simulink model "DP_GAp"  (R2023b)
settings: Solver=ode45  StartTime=0.0  StopTime=1500  RelTol=1e-3  EnableMultiTasking=on
undefined symbols (not defined in the file or in its folder): Als, Ats, Loa, pa, Ta_p
libraries: simulink x7, simulink_extras x4, marine_gnc x4, slpidlib x2
settings Model: Creator=Lenovo  LastModifiedBy=Ly Soi
settings SolverCC: AlgebraicLoopSolver=TrustRegion
settings DataIOCC: LimitDataPoints=on  SaveFormat=Array  SignalLoggingSaveFormat=ModelDataLogs  ReturnWorkspaceOutputs=off  SignalLoggingName=sigsOut
settings OptimizationCC: InitFltsAndDblsToZero=on  LifeSpan=inf
settings DebuggingCC: SaveWithParameterizedLinksMsg=none  UnderspecifiedInitializationDetection=Classic  MergeDetectMultiDrivingBlocksExec=none  SignalResolutionControl=TryResolveAllWithWarning  MultiTaskDSMMsg=warning  MultiTaskCondExecSysMsg=none  FcnCallInpInsideContextMsg=warning  UnconnectedInputMsg=warning  UnconnectedOutputMsg=warning  UnconnectedLineMsg=warning  SFUnexpectedBacktrackingDiag=warning  SFNoUnconditionalDefaultTransitionDiag=warning  ArithmeticOperatorsInVariantConditions=warning
settings HardwareCC: ProdBitPerPointer=32  ProdBitPerSizeT=32  ProdBitPerPtrDiffT=32  ProdLargestAtomicFloat=None  ProdIntDivRoundTo=Undefined  ProdEndianess=Unspecified  ProdWordSize=32  ProdHWDeviceType=32-bit Generic  TargetUnknown=on
settings ModelReferenceCC: EnableRefExpFcnMdlSchedulingChecks=on  PropagateSignalLabelsOutOfModel=off
settings SFSimCC: SimUseLocalCustomCode=off  CustomCodeUndefinedFunction=UseInterfaceOnly
settings RTWCC: RTWUseLocalCustomCode=off
settings CodeAppCC: StateflowObjectComments=on
settings GRTTargetCC: TargetFcnLib=ansi_tfl_tmw.mat  TargetLangStandard=C89/C90 (ANSI)  ModelReferenceCompliant=off  CombineOutputUpdateFcns=off  MatFileLogging=off  GRTInterface=on
settings ConfigComp: CovMetricSettings=dw  CovSaveCumulativeToWorkspaceVar=on  CovSaveSingleToWorkspaceVar=on  CovExternalEMLEnable=off  CovSFcnEnable=off

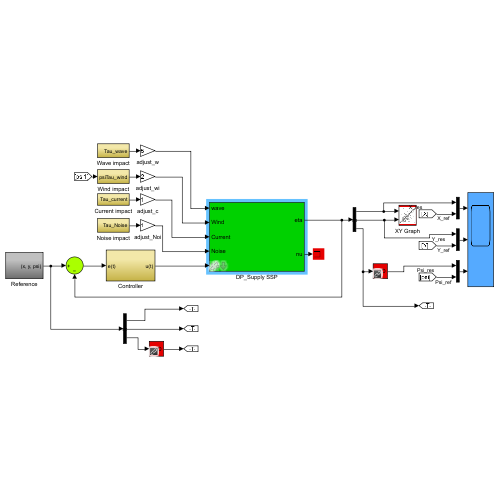
[thumbnail: Simulink's stored preview of the top-level diagram]
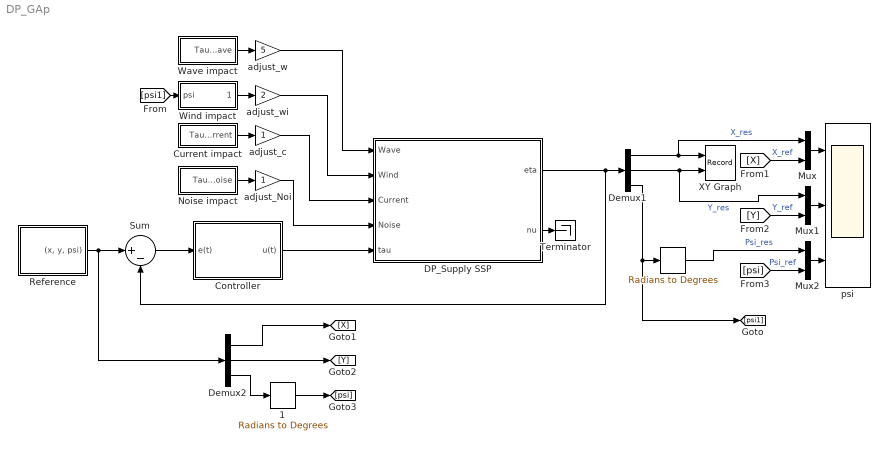
== system DP_GAp ==
  "    " : simulink_extras/Transformations/Radians to Degrees
  "    1" : simulink_extras/Transformations/Radians to Degrees
  Controller : Subsystem
  Current impact : Subsystem
  DP_Supply SSP : Subsystem  AncestorBlock=marine_gnc/Examples/Vessels/Supply vessel  mask(Supply Vessel (surge, sway and yaw)){D=[5.0242e4 0 0; 0 2.7229e5 -4.3933e6; 0 -4.3933e6 4.1894e8], Minv=inv( [5.3122e6 0 0; 0 8.2831e6 0; 0 0 3.7454e9] )}
      mask prompts: D "Linear damping matrix: D"; Minv "Inverse inertia matrix: Minv"
      mask help:
      | DP model
      |
      | Inputs:
      |
      |    tau = 3 DOF control input vector (generalized force)
      |
      | Outputs:
      |
      |    eta = [x, y, psi]'
      |    nu  = [u, v, r]'
      mask Display:
      | color('black'); port_label('output', 1, 'eta')
      | color('black'); port_label('output', 2, 'nu')
      | color('black'); port_label('input', 1, 'wave')
      | color('black'); port_label('input', 2, 'Wind')
      | color('black'); port_label('input', 3, 'Current')
      | color('black'); port_label('input', 4, 'Noise')
      | color('black'); port_label('input', 5, 'tau')
  Demux1 : Demux  Outputs=3
      settings: DisplayOption=none
  Demux2 : Demux  Outputs=3
      settings: DisplayOption=none
  Mux : Mux  Inputs=2
  Mux1 : Mux  Inputs=2
  Mux2 : Mux  Inputs=2
  Noise impact : Subsystem
  Reference : Subsystem
  Sum : Sum  Inputs=|+-
  Terminator : Terminator
  Wave impact : Subsystem
  Wind impact : Subsystem
  XY Graph : Record  FileSettingsInternal="{\"entries\":[{\"content\":{\"excelSettings\":{\"content\":{},\"type\":\"Streamout.ExcelSettings\"}},\"type\":\"Streamout.FileSettingStorage\",\"uuid\":\"\"}],\"packageUris\":[\"http:\\/\\/schema.mathworks.com\\/mf0\\/streamout_blocks\\/R2020a\"],\"version\":\"1.0\"}"  Layout=[1 1]  SignalsInternal="{\"entries\":[{\"content\":{\"signals\":[{\"content\":{\"blockPath\":[],\"dimensions\":[1],\"domain\":\"\",\"lineColor\":\"#a2142f\",\"plots\":[1],\"port\":1,\"signalID\":8,\"signalName\":\"XY Graph:1\"},\"type\":\"RecordBlkView.Signal\",\"uuid\":\"\"},{\"content\":{\"blockPath\":[],\"dimensions\":[1],\"domain\":\"\",\"lineColor\":\"#139fff\",\"plots\":[1],\"port\":2,\"signalID\":11,\"signalName\":\"XY Graph:2\"},\"type\":\"RecordBlkView.Signal\",\"uuid\":\"\"}]},\"type\":\"RecordBlkView.InputSignals\",\"uuid\":\"\"}],\"packageUris\":[\"http:\\/\\/schema.mathworks.com\\/mf0\\/streamout_blocks\\/R2020a\"],\"version\":\"1.0\"}"  VisualizationBindings="{\"xyplotplugin\":{\"info\":[{\"series\":[{\"bindingParametersList\":[{\"parameter\":\"X-Axis\",\"signalID\":8,\"signalName\":\"XY Graph:1\"},{\"parameter\":\"Y-Axis\",\"signalID\":11,\"signalName\":\"XY Graph:2\"}],\"seriesID\":17688}],\"subplotID\":1}]}}"  CompatibilityTag=XY  st=0.1
  adjust_Noi : Gain
  adjust_c : Gain
  adjust_w : Gain  Gain=5
  adjust_wi : Gain  Gain=2
  psi : Scope  NumInputPorts=3
  wires:
  Reference/1("(x, y, psi)") -> Demux2/1, Sum/1
  Sum/1 -> Controller/1(e(t))
  DP_Supply SSP/2(nu) -> Terminator/1
  Demux1/1 -> Mux/1, XY Graph/1  "X_res"
  Demux1/2 -> Mux1/1, XY Graph/2  "Y_res"
  DP_Supply SSP/1(eta) -> Sum/2, Demux1/1
  Demux1/3 -> "    "/1, [psi1]
  Controller/1(u(t)) -> DP_Supply SSP/5(tau)
  Mux/1 -> psi/1
  [X] -> Mux/2  "X_ref"
  Demux2/1 -> [X]
  Mux1/1 -> psi/2
  [Y] -> Mux1/2  "Y_ref"
  Demux2/2 -> [Y]
  Mux2/1 -> psi/3
  [psi] -> Mux2/2  "Psi_ref"
  "    "/1 -> Mux2/1  "Psi_res"
  Demux2/3 -> "    1"/1
  "    1"/1 -> [psi]
  Current impact/1(Tau_current) -> adjust_c/1
  Wave impact/1(Tau_wave) -> adjust_w/1
  Noise impact/1(Tau_Noise) -> adjust_Noi/1
  Wind impact/1(Tau_wind) -> adjust_wi/1
  [psi1] -> Wind impact/1(psi)
  adjust_Noi/1 -> DP_Supply SSP/4(Noise)
  adjust_c/1 -> DP_Supply SSP/3(Current)
  adjust_wi/1 -> DP_Supply SSP/2(Wind)
  adjust_w/1 -> DP_Supply SSP/1(Wave)

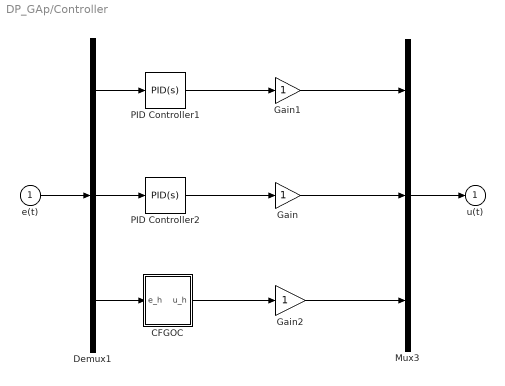
== system DP_GAp/Controller ==
  e(t) : Inport
  CFGOC : Subsystem
  Demux1 : Demux  Outputs=3
  Gain : Gain
  Gain1 : Gain
  Gain2 : Gain
  Mux3 : Mux  Inputs=3
  PID Controller1 : slpidlib/PID Controller  Controller=PID  Form=Parallel  TimeDomain=Continuous-time  UseExternalTs=off  SampleTime=-1  IntegratorMethod=Forward Euler  FilterMethod=Forward Euler  ControllerParametersSource=internal  P=13982.7626612688  I=79.4713079858411  UseKiTs=off  D=614214.172913347  N=13.3180631687176  UseFilter=on  TunerSelectOption=Transfer Function Based (PID Tuner App)  InitialConditionSource=internal  InitialConditionForIntegrator=0  InitialConditionForFilter=0  DifferentiatorICPrevScaledInput=0  ExternalReset=none  TrackingMode=off  Kt=1  LimitOutput=off  SatLimitsSource=internal  UpperSaturationLimit=inf  LowerSaturationLimit=-inf  LinearizeAsGain=on  AntiWindupMode=none  Kb=1  LimitIntegrator=off  UpperIntegratorSaturationLimit=inf  LowerIntegratorSaturationLimit=-inf  POutMin=[]  POutMax=[]  IOutMin=[]  IOutMax=[]  DOutMin=[]  DOutMax=[]  NOutMin=[]  NOutMax=[]  SumOutMin=[]  SumOutMax=[]  SaturationOutMin=[]  SaturationOutMax=[]  PParamMin=[]  PParamMax=[]  IParamMin=[]  IParamMax=[]  DParamMin=[]  DParamMax=[]  NParamMin=[]  NParamMax=[]  KbParamMin=[]  KbParamMax=[]  KtParamMin=[]  KtParamMax=[]  KbOutMin=[]  KbOutMax=[]  KtOutMin=[]  KtOutMax=[]  IntegratorOutMin=[]  IntegratorOutMax=[]  FilterOutMin=[]  FilterOutMax=[]  SumI1OutMin=[]  SumI1OutMax=[]  SumI2OutMin=[]  SumI2OutMax=[]  SumI3OutMin=[]  SumI3OutMax=[]  SumI4OutMin=[]  SumI4OutMax=[]  SumDOutMin=[]  SumDOutMax=[]  DifferentiatorOutMin=[]  DifferentiatorOutMax=[]  FilterDiffOutCoefMin=[]  FilterDiffOutCoefMax=[]  ReciprocalOutMin=[]  ReciprocalOutMax=[]  SumDenOutMin=[]  SumDenOutMax=[]  SumNumOutMin=[]  SumNumOutMax=[]  DivideOutMin=[]  DivideOutMax=[]  UdiffTsProdOutMin=[]  UdiffTsProdOutMax=[]  NTsProdOutMin=[]  NTsProdOutMax=[]  UintegralTsProdOutMin=[]  UintegralTsProdOutMax=[]  UngainTsProdOutMin=[]  UngainTsProdOutMax=[]  ClampingZeroOutDataTypeStr=Inherit: Inherit via back propagation  ClampingZeroOutMin=[]  ClampingZeroOutMax=[]  FilterDenConstantOutDataTypeStr=Inherit: Inherit via back propagation  FilterDenConstantOutMin=[]  FilterDenConstantOutMax=[]  PCopyOutDataTypeStr=Inherit: Inherit via back propagation  PCopyOutMin=[]  PCopyOutMax=[]  NCopyOutDataTypeStr=Inherit: Inherit via back propagation  NCopyOutMin=[]  NCopyOutMax=[]  IntegratorContinuousStateAttributes=''  IntegratorStateMustResolveToSignalObject=off  IntegratorRTWStateStorageClass=Auto  FilterContinuousStateAttributes=''  FilterStateMustResolveToSignalObject=off  FilterRTWStateStorageClass=Auto  ParallelPVariant=InternalParameters  IdealPVariant=Disabled  IVariant=InternalParameters  DVariant=InternalParameters  IntegratorVariant=Continuous  SatVariant=Disabled  AWVariant=Passthrough  PCopyVariant=Disabled  TRVariant=Disabled  FdbkBlocksVariant=Forward  IdealPFdbkVariant=Disabled  SatFdbkVariant=Disabled  DerivativeFilterVariant=ContFilter  NVariant=InternalParameters  NCopyVariant=Disabled  FilterICVariant=InternalICsFilter  IntegratorICVariant=InternalICs  ExternalResetVariant=Disabled  TRSumVariant=Passthrough  SumFdbkVariant=Disabled  SumVariant=Sum_PID  TsampFilterVariant=InternalTs  TsampNgainVariant=Passthrough  TsampIntegralVariant=Disabled_SignalSpec  ExternalSaturationOutDataTypeStr=Inherit: Same as second input
  PID Controller2 : slpidlib/PID Controller  Controller=PID  Form=Parallel  TimeDomain=Continuous-time  UseExternalTs=off  SampleTime=-1  IntegratorMethod=Forward Euler  FilterMethod=Forward Euler  ControllerParametersSource=internal  P=330751.15042107  I=6499.51593881031  UseKiTs=off  D=3225830.41285156  N=4.23253792984163  UseFilter=on  TunerSelectOption=Transfer Function Based (PID Tuner App)  InitialConditionSource=internal  InitialConditionForIntegrator=0  InitialConditionForFilter=0  DifferentiatorICPrevScaledInput=0  ExternalReset=none  TrackingMode=off  Kt=1  LimitOutput=off  SatLimitsSource=internal  UpperSaturationLimit=inf  LowerSaturationLimit=-inf  LinearizeAsGain=on  AntiWindupMode=none  Kb=1  LimitIntegrator=off  UpperIntegratorSaturationLimit=inf  LowerIntegratorSaturationLimit=-inf  POutMin=[]  POutMax=[]  IOutMin=[]  IOutMax=[]  DOutMin=[]  DOutMax=[]  NOutMin=[]  NOutMax=[]  SumOutMin=[]  SumOutMax=[]  SaturationOutMin=[]  SaturationOutMax=[]  PParamMin=[]  PParamMax=[]  IParamMin=[]  IParamMax=[]  DParamMin=[]  DParamMax=[]  NParamMin=[]  NParamMax=[]  KbParamMin=[]  KbParamMax=[]  KtParamMin=[]  KtParamMax=[]  KbOutMin=[]  KbOutMax=[]  KtOutMin=[]  KtOutMax=[]  IntegratorOutMin=[]  IntegratorOutMax=[]  FilterOutMin=[]  FilterOutMax=[]  SumI1OutMin=[]  SumI1OutMax=[]  SumI2OutMin=[]  SumI2OutMax=[]  SumI3OutMin=[]  SumI3OutMax=[]  SumI4OutMin=[]  SumI4OutMax=[]  SumDOutMin=[]  SumDOutMax=[]  DifferentiatorOutMin=[]  DifferentiatorOutMax=[]  FilterDiffOutCoefMin=[]  FilterDiffOutCoefMax=[]  ReciprocalOutMin=[]  ReciprocalOutMax=[]  SumDenOutMin=[]  SumDenOutMax=[]  SumNumOutMin=[]  SumNumOutMax=[]  DivideOutMin=[]  DivideOutMax=[]  UdiffTsProdOutMin=[]  UdiffTsProdOutMax=[]  NTsProdOutMin=[]  NTsProdOutMax=[]  UintegralTsProdOutMin=[]  UintegralTsProdOutMax=[]  UngainTsProdOutMin=[]  UngainTsProdOutMax=[]  ClampingZeroOutDataTypeStr=Inherit: Inherit via back propagation  ClampingZeroOutMin=[]  ClampingZeroOutMax=[]  FilterDenConstantOutDataTypeStr=Inherit: Inherit via back propagation  FilterDenConstantOutMin=[]  FilterDenConstantOutMax=[]  PCopyOutDataTypeStr=Inherit: Inherit via back propagation  PCopyOutMin=[]  PCopyOutMax=[]  NCopyOutDataTypeStr=Inherit: Inherit via back propagation  NCopyOutMin=[]  NCopyOutMax=[]  IntegratorContinuousStateAttributes=''  IntegratorStateMustResolveToSignalObject=off  IntegratorRTWStateStorageClass=Auto  FilterContinuousStateAttributes=''  FilterStateMustResolveToSignalObject=off  FilterRTWStateStorageClass=Auto  ParallelPVariant=InternalParameters  IdealPVariant=Disabled  IVariant=InternalParameters  DVariant=InternalParameters  IntegratorVariant=Continuous  SatVariant=Disabled  AWVariant=Passthrough  PCopyVariant=Disabled  TRVariant=Disabled  FdbkBlocksVariant=Forward  IdealPFdbkVariant=Disabled  SatFdbkVariant=Disabled  DerivativeFilterVariant=ContFilter  NVariant=InternalParameters  NCopyVariant=Disabled  FilterICVariant=InternalICsFilter  IntegratorICVariant=InternalICs  ExternalResetVariant=Disabled  TRSumVariant=Passthrough  SumFdbkVariant=Disabled  SumVariant=Sum_PID  TsampFilterVariant=InternalTs  TsampNgainVariant=Passthrough  TsampIntegralVariant=Disabled_SignalSpec  ExternalSaturationOutDataTypeStr=Inherit: Same as second input
  u(t) : Outport
  wires:
  Mux3/1 -> u(t)/1
  Demux1/2 -> PID Controller2/1
  Demux1/3 -> CFGOC/1(e_h)
  e(t)/1 -> Demux1/1
  Gain/1 -> Mux3/2
  Gain2/1 -> Mux3/3
  CFGOC/1(u_h) -> Gain2/1
  Demux1/1 -> PID Controller1/1
  Gain1/1 -> Mux3/1
  PID Controller2/1 -> Gain/1
  PID Controller1/1 -> Gain1/1

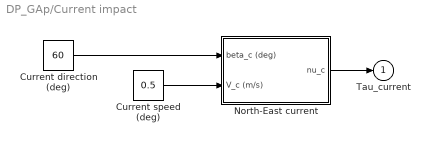
== system DP_GAp/Current impact ==
  Current direction (deg) : Constant  Value=60
  Current speed (deg) : Constant  Value=0.5
  North-East current : Subsystem  AncestorBlock=marine_gnc/Environment/Current/North-East current
  Tau_current : Outport
  wires:
  Current speed (deg)/1 -> North-East current/2(V_c (m/s))
  Current direction (deg)/1 -> North-East current/1(beta_c (deg))
  North-East current/1(nu_c) -> Tau_current/1

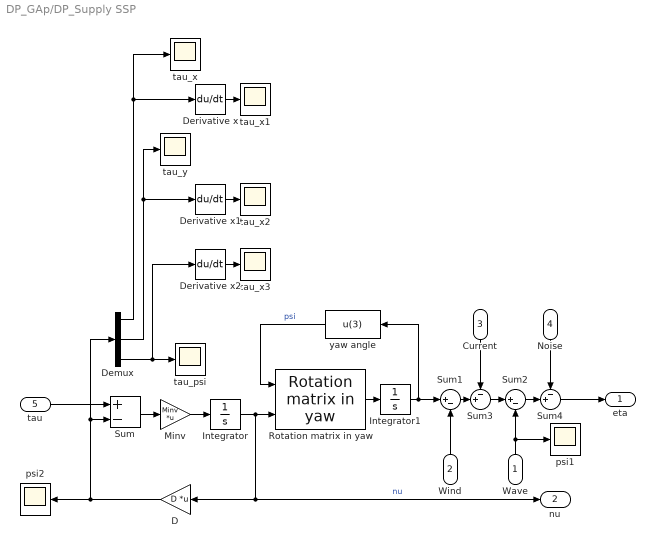
== system DP_GAp/DP_Supply SSP ==
  Wave : Inport
  Wind : Inport  Port=2
  Current : Inport  Port=3
  Noise : Inport  Port=4
  tau : Inport  Port=5
  D : Gain  Gain=D  Multiplication=Matrix(K*u)  SaturateOnIntegerOverflow=on  OutDataTypeStr=Inherit: Same as input  ParamDataTypeStr=Inherit: Same as input
  Demux : Demux  Outputs=3
  Derivative x : Derivative
  Derivative x1 : Derivative
  Derivative x2 : Derivative
  Integrator : Integrator
  Integrator1 : Integrator
  Minv : Gain  Gain=Minv  Multiplication=Matrix(K*u)  SaturateOnIntegerOverflow=on  OutDataTypeStr=Inherit: Same as input  ParamDataTypeStr=Inherit: Same as input
  "Rotation matrix in yaw " : marine_gnc/Models/ Kinematics/Rotation matrix in yaw 
  Sum : Sum  Inputs=+-  InputSameDT=on  SaturateOnIntegerOverflow=on  OutDataTypeStr=Inherit: Same as first input
  Sum1 : Sum  Inputs=|+-
  Sum2 : Sum  Inputs=|+-
  Sum3 : Sum  Inputs=-+|
  Sum4 : Sum  Inputs=-+|
  psi1 : Scope
  psi2 : Scope
  tau_psi : Scope
  tau_x{,1..3} (4 alike) : Scope
  tau_y : Scope
  yaw angle : Fcn  Expr=u(3)
  eta : Outport  InitialOutput=0
  nu : Outport  Port=2  InitialOutput=0
  wires:
  D/1 -> Demux/1, Sum/2, psi2/1
  Sum/1 -> Minv/1
  Minv/1 -> Integrator/1
  "Rotation matrix in yaw "/1 -> Integrator1/1
  yaw angle/1 -> "Rotation matrix in yaw "/1  "psi"
  Integrator/1 -> nu/1, D/1, "Rotation matrix in yaw "/2  "nu"
  Wind/1 -> Sum1/2
  Wave/1 -> Sum2/2, psi1/1
  Integrator1/1 -> Sum1/1, yaw angle/1
  tau/1 -> Sum/1
  Demux/1 -> Derivative x/1, tau_x/1
  Demux/2 -> Derivative x1/1, tau_y/1
  Derivative x/1 -> tau_x1/1
  Derivative x1/1 -> tau_x2/1
  Demux/3 -> Derivative x2/1, tau_psi/1
  Derivative x2/1 -> tau_x3/1
  Sum4/1 -> eta/1
  Current/1 -> Sum3/1
  Sum1/1 -> Sum3/2
  Sum3/1 -> Sum2/1
  Sum2/1 -> Sum4/2
  Noise/1 -> Sum4/1

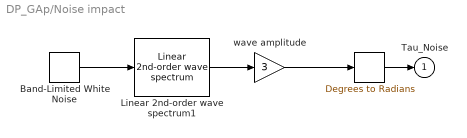
== system DP_GAp/Noise impact ==
  "   " : simulink_extras/Transformations/Degrees to Radians
  Band-Limited White Noise : simulink/Sources/Band-Limited White Noise  Cov=[1]  Ts=0.1  seed=[23341]
  Linear 2nd-order wave spectrum1 : marine_gnc/Environment/Waves/Linear 2nd-order  wave spectrum  sigma=.5  w_0=1.2  lambda=0.1
  wave amplitude : Gain  Gain=3  SaturateOnIntegerOverflow=on  OutDataTypeStr=Inherit: Same as input  ParamDataTypeStr=Inherit: Same as input
  Tau_Noise : Outport
  wires:
  "   "/1 -> Tau_Noise/1
  Band-Limited White Noise/1 -> Linear 2nd-order wave spectrum1/1
  Linear 2nd-order wave spectrum1/1 -> wave amplitude/1
  wave amplitude/1 -> "   "/1

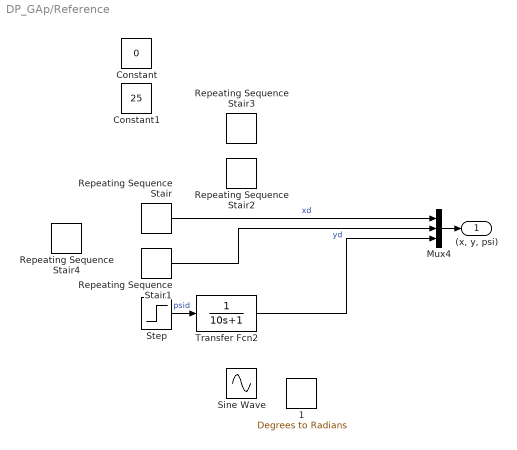
== system DP_GAp/Reference ==
  "     1" : simulink_extras/Transformations/Degrees to Radians
  Constant : Constant  Value=0
  Constant1 : Constant  Value=25
  Mux4 : Mux  Inputs=3
  Repeating Sequence Stair : simulink/Sources/Repeating Sequence Stair  OutValues=[-3 -7 0 7]  tsamp=300  OutMin=[]  OutMax=[]  OutDataTypeStr=double  OutputDataTypeScalingMode=double  OutDataType=fixdt(0,8)  ConRadixGroup=Best Precision: Vector-wise  OutScaling=2^-12
  Repeating Sequence Stair1 : simulink/Sources/Repeating Sequence Stair  OutValues=[-7 0 7 0]  tsamp=300  OutMin=[]  OutMax=[]  OutDataTypeStr=double  OutputDataTypeScalingMode=double  OutDataType=fixdt(0,8)  ConRadixGroup=Best Precision: Vector-wise  OutScaling=2^-12
  Repeating Sequence Stair2 : simulink/Sources/Repeating Sequence Stair  OutValues=[7 -7 0 7]  tsamp=0.2  OutMin=[]  OutMax=[]  OutDataTypeStr=double  OutputDataTypeScalingMode=double  OutDataType=fixdt(0,8)  ConRadixGroup=Best Precision: Vector-wise  OutScaling=2^-12
  Repeating Sequence Stair3 : simulink/Sources/Repeating Sequence Stair  OutValues=[-7 7 0 7]  tsamp=0.2  OutMin=[]  OutMax=[]  OutDataTypeStr=double  OutputDataTypeScalingMode=double  OutDataType=fixdt(0,8)  ConRadixGroup=Best Precision: Vector-wise  OutScaling=2^-12
  Repeating Sequence Stair4 : simulink/Sources/Repeating Sequence Stair  OutValues=[7 -7 0 7]  tsamp=0.2  OutMin=[]  OutMax=[]  OutDataTypeStr=double  OutputDataTypeScalingMode=double  OutDataType=fixdt(0,8)  ConRadixGroup=Best Precision: Vector-wise  OutScaling=2^-12
  Sine Wave : Sin  Amplitude=20  Frequency=10  SampleTime=0
  Step : Step  Time=0  After=20  SampleTime=0
  Transfer Fcn2 : TransferFcn  Denominator=[10 1]
  "(x, y, psi)" : Outport
  wires:
  Mux4/1 -> "(x, y, psi)"/1
  Step/1 -> Transfer Fcn2/1  "psid"
  Repeating Sequence Stair1/1 -> Mux4/2  "yd"
  Repeating Sequence Stair/1 -> Mux4/1  "xd"
  Transfer Fcn2/1 -> Mux4/3

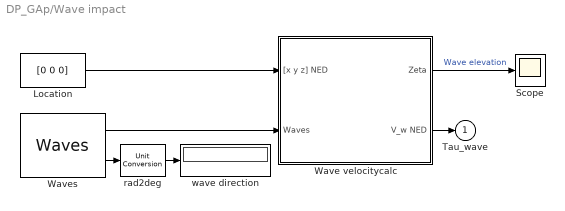
== system DP_GAp/Wave impact ==
  Location : Constant  Value=[0 0 0]
  Scope : Scope
  Wave velocitycalc : Subsystem  AncestorBlock=marine_gnc/Environment/Waves/Wave velocitycalc  mask(Wave velocitycalc){}
      mask help: Caclulates the wave-induced water velocity in NED coordinates and surface elevation Zeta at the point [x y z] in NED. The Waves bus generated by the Waves module is needed as input.
  Waves : marine_gnc/Environment/Waves/Waves  spectrum_type=ITTC  disp_flag=off  plot_spectrum=off  plot_realization=off  hs=0.8  omega_peak=0  psi_mean=0  gamma=-1  spread=2  depth=inf  nfreq=20  ndir=10  energylim=0.005  freq_cutoff=3  dir_cutoff=0  rand_seed=123  rand_freq=on  rand_dir=on  Zeta_a=0  Omega=0  Phase=0  Wavenum=0  Psi=0
  rad2deg : marine_gnc/Utilities/Math Operations/Unit Conversion  in=rad2deg
  wave direction : Display
  Tau_wave : Outport
  wires:
  Waves/1 -> Wave velocitycalc/2(Waves)
  Location/1 -> Wave velocitycalc/1("[x y z] NED")
  Wave velocitycalc/1(Zeta) -> Scope/1  "Wave elevation"
  Waves/2 -> rad2deg/1
  rad2deg/1 -> wave direction/1
  Wave velocitycalc/2(V_w NED) -> Tau_wave/1

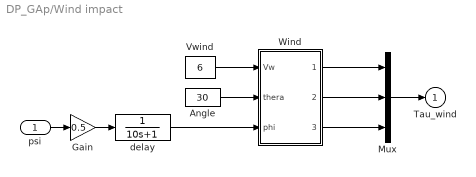
== system DP_GAp/Wind impact ==
  psi : Inport
  Angle : Constant  Value=30
  Gain : Gain  Gain=0.5
  Mux : Mux  Inputs=3
  Vwind : Constant  Value=6
  Wind : Subsystem
  delay : TransferFcn  Denominator=[10 1]
  Tau_wind : Outport
  wires:
  Mux/1 -> Tau_wind/1
  Angle/1 -> Wind/2(thera)
  Vwind/1 -> Wind/1(Vw)
  Wind/1(Xwind) -> Mux/1
  Wind/2(Ywind) -> Mux/2
  Wind/3(Nwind) -> Mux/3
  psi/1 -> Gain/1
  Gain/1 -> delay/1
  delay/1 -> Wind/3(phi)

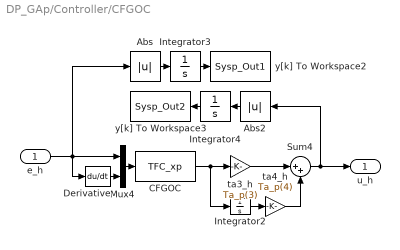
== system DP_GAp/Controller/CFGOC ==
  e_h : Inport
  Abs : Abs  SaturateOnIntegerOverflow=off
  Abs2 : Abs  SaturateOnIntegerOverflow=off
  CFGOC : MATLABFcn  MATLABFcn=TFC_xp  OutputDimensions=1
  Derivative : Derivative
  Integrator2 : Integrator
  Integrator3 : Integrator
  Integrator4 : Integrator
  Mux4 : Mux  Inputs=2
  Sum4 : Sum  Inputs=|++  InputSameDT=on  SaturateOnIntegerOverflow=on  OutDataTypeStr=Inherit: Same as first input
  ta3_h : Gain  Gain=Ta_p(3)
  ta4_h : Gain  Gain=Ta_p(4)
  y[k] To Workspace2 : ToWorkspace  VariableName=Sysp_Out1  SaveFormat=Timeseries  SampleTime=-1
  y[k] To Workspace3 : ToWorkspace  VariableName=Sysp_Out2  SaveFormat=Timeseries  SampleTime=-1
  u_h : Outport
  wires:
  Sum4/1 -> u_h/1, Abs2/1
  Derivative/1 -> Mux4/2
  Mux4/1 -> CFGOC/1
  CFGOC/1 -> ta3_h/1, Integrator2/1
  Integrator2/1 -> ta4_h/1
  ta4_h/1 -> Sum4/2
  ta3_h/1 -> Sum4/1
  e_h/1 -> Abs/1, Derivative/1, Mux4/1
  Integrator3/1 -> y[k] To Workspace2/1
  Integrator4/1 -> y[k] To Workspace3/1
  Abs/1 -> Integrator3/1
  Abs2/1 -> Integrator4/1

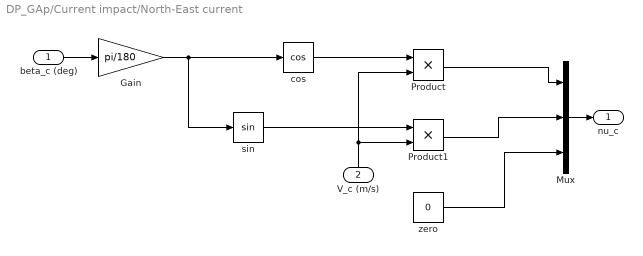
== system DP_GAp/Current impact/North-East current ==
  beta_c (deg) : Inport
  V_c (m/s) : Inport  Port=2
  Gain : Gain  Gain=pi/180
  Mux : Mux  Inputs=3
  Product : Product  RndMeth=Zero
  Product1 : Product  RndMeth=Zero
  cos : Trigonometry  Operator=cos
  sin : Trigonometry
  zero : Constant  Value=0
  nu_c : Outport
  wires:
  Mux/1 -> nu_c/1
  beta_c (deg)/1 -> Gain/1
  zero/1 -> Mux/3
  Product1/1 -> Mux/2
  Product/1 -> Mux/1
  sin/1 -> Product1/1
  V_c (m/s)/1 -> Product/2, Product1/2
  cos/1 -> Product/1
  Gain/1 -> cos/1, sin/1

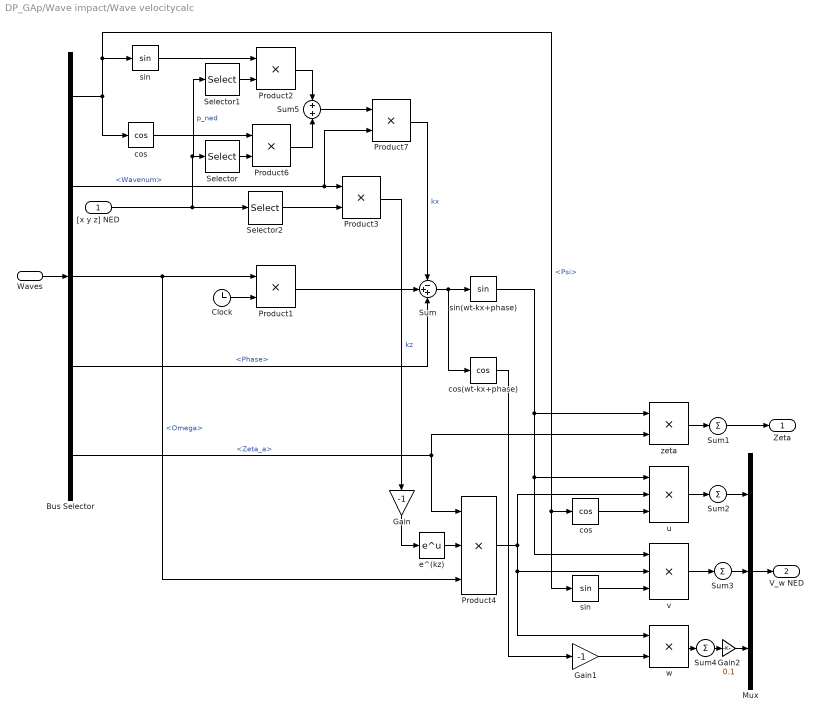
== system DP_GAp/Wave impact/Wave velocitycalc ==
  "[x y z] NED" : Inport
  Waves : Inport  Port=2
  Bus Selector : BusSelector  OutputSignals=Psi,Wavenum,Omega,Phase,Zeta_a
  Clock : Clock
  Gain : Gain  Gain=-1  SaturateOnIntegerOverflow=on  OutDataTypeStr=Inherit: Same as input  ParamDataTypeStr=Inherit: Same as input
  Gain1 : Gain  Gain=-1  SaturateOnIntegerOverflow=on  OutDataTypeStr=Inherit: Same as input  ParamDataTypeStr=Inherit: Same as input
  Gain2 : Gain  Gain=0.1  SaturateOnIntegerOverflow=on  OutDataTypeStr=Inherit: Same as input  ParamDataTypeStr=Inherit: Same as input
  Mux : Mux  Inputs=3
  Product{1..3,6..7} (5 alike) : Product  Inputs=**  SaturateOnIntegerOverflow=on  OutDataTypeStr=Inherit: Same as first input
  Product4 : Product  Inputs=3  SaturateOnIntegerOverflow=on  OutDataTypeStr=Inherit: Same as first input
  Selector : Selector  InputPortWidth=3  IndexOptions=Index vector (dialog)  Indices=1  OutputSizes=1
  Selector1 : Selector  InputPortWidth=3  IndexOptions=Index vector (dialog)  Indices=2  OutputSizes=1
  Selector2 : Selector  InputPortWidth=3  IndexOptions=Index vector (dialog)  Indices=3  OutputSizes=1
  Sum : Sum  Inputs=-++  SaturateOnIntegerOverflow=on
  Sum{1..4} (4 alike) : Sum  Inputs=1  SaturateOnIntegerOverflow=on
  Sum5 : Sum  SaturateOnIntegerOverflow=on
  cos : Trigonometry  Operator=cos
  "cos " : Trigonometry  Operator=cos
  cos(wt-kx+phase) : Trigonometry  Operator=cos
  e^(kz) : Math  SignedPower=on
  sin : Trigonometry
  "sin " : Trigonometry
  sin(wt-kx+phase) : Trigonometry
  u : Product  Inputs=***  SaturateOnIntegerOverflow=on  OutDataTypeStr=Inherit: Same as first input
  v : Product  Inputs=***  SaturateOnIntegerOverflow=on  OutDataTypeStr=Inherit: Same as first input
  w : Product  Inputs=**  SaturateOnIntegerOverflow=on  OutDataTypeStr=Inherit: Same as first input
  zeta : Product  Inputs=**  SaturateOnIntegerOverflow=on  OutDataTypeStr=Inherit: Same as first input
  Zeta : Outport
  V_w NED : Outport  Port=2
  wires:
  Clock/1 -> Product1/2
  Mux/1 -> V_w NED/1
  Sum3/1 -> Mux/2
  Sum2/1 -> Mux/1
  v/1 -> Sum3/1
  u/1 -> Sum2/1
  w/1 -> Sum4/1
  Sum1/1 -> Zeta/1
  Product3/1 -> Gain/1  "kz"
  Bus Selector/1 -> sin/1, "sin "/1, "cos "/1, cos/1  "<Psi>"
  Product1/1 -> Sum/2
  Sum/1 -> sin(wt-kx+phase)/1, cos(wt-kx+phase)/1
  sin(wt-kx+phase)/1 -> zeta/1, u/1, v/1
  zeta/1 -> Sum1/1
  Product7/1 -> Sum/1  "kx"
  e^(kz)/1 -> Product4/2
  Product4/1 -> u/2, v/2, w/1
  cos(wt-kx+phase)/1 -> Gain1/1
  Waves/1 -> Bus Selector/1
  Bus Selector/3 -> Product1/1, Product4/3  "<Omega>"
  Bus Selector/4 -> Sum/3  "<Phase>"
  Bus Selector/5 -> zeta/2, Product4/1  "<Zeta_a>"
  Gain/1 -> e^(kz)/1
  Bus Selector/2 -> Product7/2, Product3/1  "<Wavenum>"
  Selector/1 -> Product6/2
  cos/1 -> Product6/1
  Selector1/1 -> Product2/2
  sin/1 -> Product2/1
  Product2/1 -> Sum5/1
  Product6/1 -> Sum5/2
  Sum5/1 -> Product7/1
  "[x y z] NED"/1 -> Selector2/1, Selector1/1, Selector/1  "p_ned"
  Selector2/1 -> Product3/2
  "sin "/1 -> v/3
  "cos "/1 -> u/3
  Gain1/1 -> w/2
  Sum4/1 -> Gain2/1
  Gain2/1 -> Mux/3

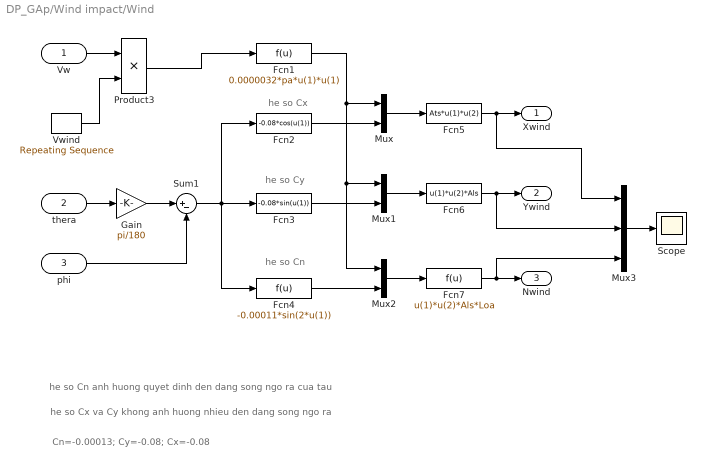
== system DP_GAp/Wind impact/Wind ==
  note: he so Cy
  note: he so Cn
  note: he so Cx
  note: he so Cn anh huong quyet dinh den dang song ngo ra cua tau
  note: he so Cx va Cy khong anh huong nhieu den dang song ngo ra
  note: Cn=-0.00013; Cy=-0.08; Cx=-0.08
  Vw : Inport
  thera : Inport  Port=2
  phi : Inport  Port=3
  Fcn1 : Fcn  Expr=0.0000032*pa*u(1)*u(1)
  Fcn2 : Fcn  Expr=-0.08*cos(u(1))
  Fcn3 : Fcn  Expr=-0.08*sin(u(1))
  Fcn4 : Fcn  Expr=-0.00011*sin(2*u(1))
  Fcn5 : Fcn  Expr=Ats*u(1)*u(2)
  Fcn6 : Fcn  Expr=u(1)*u(2)*Als
  Fcn7 : Fcn  Expr=u(1)*u(2)*Als*Loa
  Gain : Gain  Gain=pi/180
  Mux : Mux  Inputs=2
  Mux1 : Mux  Inputs=2
  Mux2 : Mux  Inputs=2
  Mux3 : Mux  Inputs=3
  Product3 : Product  RndMeth=Zero
  Scope : Scope
  Sum1 : Sum  Inputs=|+-
  Vwind : simulink/Sources/Repeating Sequence  rep_seq_t=[0 500 510 530 550 900 910 930 950 1100]  rep_seq_y=[0 0 1 1 0 0 1 1 0 0]
  Xwind : Outport
  Ywind : Outport  Port=2
  Nwind : Outport  Port=3
  wires:
  phi/1 -> Sum1/2
  Fcn1/1 -> Mux/1, Mux1/1, Mux2/1
  Mux/1 -> Fcn5/1
  Fcn5/1 -> Xwind/1, Mux3/1
  Mux1/1 -> Fcn6/1
  Mux2/1 -> Fcn7/1
  Fcn6/1 -> Ywind/1, Mux3/2
  Fcn7/1 -> Nwind/1, Mux3/3
  Gain/1 -> Sum1/1
  thera/1 -> Gain/1
  Sum1/1 -> Fcn3/1, Fcn2/1, Fcn4/1
  Fcn2/1 -> Mux/2
  Fcn3/1 -> Mux1/2
  Fcn4/1 -> Mux2/2
  Mux3/1 -> Scope/1
  Vw/1 -> Product3/1
  Product3/1 -> Fcn1/1
  Vwind/1 -> Product3/2
